simulink model "IP_Sim"  (R2022a)
settings: Solver=FixedStepAuto  StartTime=0.0  StopTime=inf  FixedStep=0.01  RelTol=1e-3
InitFcn:
  | M = 0.5;
  | m = 0.5;
  | l = 0.3;
  | I = 0.006;
  | mu = 0.1;
  | g = 9.81
libraries: vrlib x2
settings Model: Creator=jitendra  LastModifiedBy=vcichella
settings DataIOCC: ExternalInput=getinputstruct(op_trim1)  InitialState=getstatestruct(op_trim1)  ReturnWorkspaceOutputs=off
settings DebuggingCC: UnconnectedInputMsg=warning  UnconnectedOutputMsg=warning  UnconnectedLineMsg=warning  SFMachineParentedDataDiag=warning  ArithmeticOperatorsInVariantConditions=warning
settings SFSimCC: SimUseLocalCustomCode=off  CustomCodeUndefinedFunction=UseInterfaceOnly
settings RTWCC: RTWUseLocalCustomCode=off

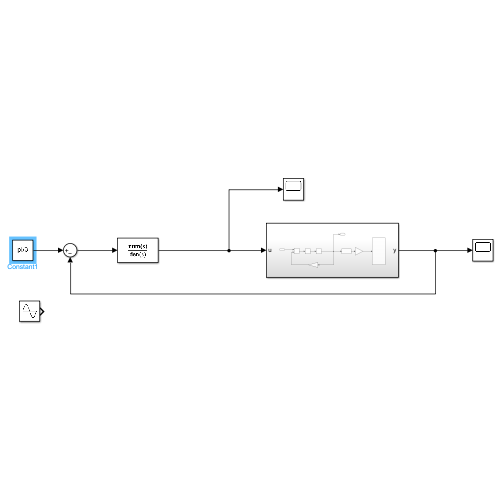
[thumbnail: Simulink's stored preview of the top-level diagram]
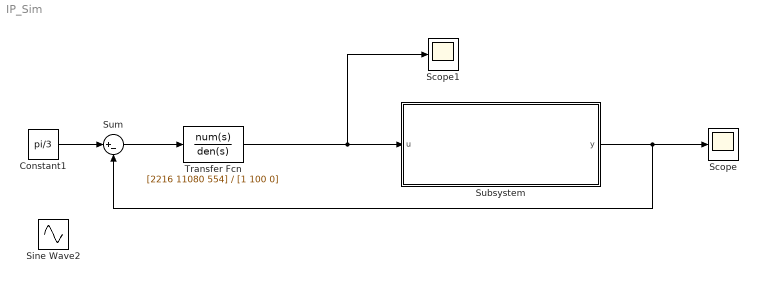
== system IP_Sim ==
  Constant1 : Constant  Value=pi/3
  Scope : Scope
  Scope1 : Scope
  Sine Wave2 : Sin  Amplitude=0.1  Frequency=0.5  SampleTime=0
  Subsystem : Subsystem
  Sum : Sum  Inputs=|+-
  Transfer Fcn : TransferFcn  Numerator=[2216 11080 554]  Denominator=[1 100 0]
  wires:
  Sum/1 -> Transfer Fcn/1
  Subsystem/1(y) -> Scope/1, Sum/2
  Transfer Fcn/1 -> Scope1/1, Subsystem/1(u)
  Constant1/1 -> Sum/1

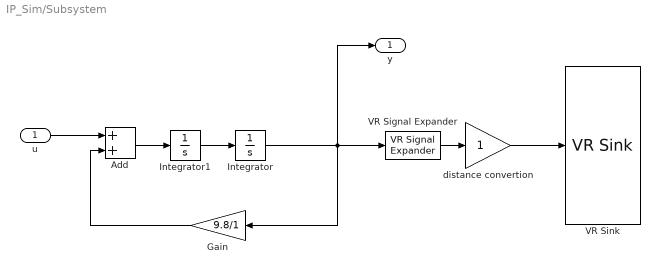
== system IP_Sim/Subsystem ==
  u : Inport
  Add : Sum
  Gain : Gain  Gain=9.8/1
  Integrator : Integrator
  Integrator1 : Integrator
  VR Signal Expander : vrlib/VR Signal Expander  outwidth=4  outidx=[4]
  VR Sink : vrlib/VR Sink  InstantiateOnLoad=on  SampleTime=0.02  ViewEnable=on  RemoteChange=off  RemoteView=off  FieldsWritten=joint.rotation.4.1.1.double  WorldFileName=InvertedPendulum.wrl  AutoView=on  VideoDimensions=[]  AllowVariableSize=off  FigureProperties="{'Position', 'Name', 'Viewpoint', 'CameraBound', 'CameraDirection', 'CameraPosition', 'CameraUpVector', 'ZoomFactor', 'Antialiasing', 'Headlight', 'Lighting', 'NavPanel', 'Sound', 'StatusBar', 'Stereo3D', 'Stereo3DCameraOffset', 'Stereo3DHIT', 'ToolBar', 'Textures', 'Transparency', 'Triad', 'Wireframe', 'NavZones', 'NavMode', 'NavSpeed', 'CaptureFileFormat', 'CaptureFileName', 'Record2DCompressMethod', 'Record2DCompressQuality', 'Record2D', 'Record2DFileName', 'Record2DFPS'; [1.9210000000000000e+03   7.6000000000000000e+01   1.9200000000000000e+03   9.1300000000000000e+02], '', '', 'on', [0.0000000000000000e+00   0.0000000000000000e+00  -1.0000000000000000e+00], [0.0000000000000000e+00   0.0000000000000000e+00   1.4153853988647461e+01], [0.0000000000000000e+00   1.0000000000000000e+00   0.0000000000000000e+00], [1.0000000000000000e+00], 'on', 'on', 'on', 'halfbar', 'on', 'on', 'off', [1.0000000149011612e-01], [0.0000000000000000e+00], 'on', 'on', 'on', 'none', 'off', 'off', 'fly', 'normal', 'tif', '%f_anim_%n.tif', 'auto', [7.5000000000000000e+01], 'off', '%f_anim_%n.avi', 'auto'}"
  distance convertion : Gain
  y : Outport
  wires:
  Add/1 -> Integrator1/1
  Integrator/1 -> y/1, Gain/1, VR Signal Expander/1
  u/1 -> Add/1
  Integrator1/1 -> Integrator/1
  Gain/1 -> Add/2
  VR Signal Expander/1 -> distance convertion/1
  distance convertion/1 -> VR Sink/1
